simulink model "VehCtrl20260630_18B"  (R2018b)
settings: Solver=FixedStepAuto  StartTime=0.0  StopTime=inf  FixedStep=0.005  RelTol=1e-3
InitFcn:
  | mbd_mpc_consistency_checks(bdroot(gcs));
undefined symbols (not defined in the file): ANG_DEAD, BMS_NormalPwr, BrakeDeadZone, BrkPrsByBrkPct_TB_X, BrkPrsByBrkPct_TB_Y, DELAY_DISCHARGE, DELAY_RCUOFF, DRV_BACKWARD, DRV_BRAKE, DRV_FORWARD, DRV_NEUTRAL, DRV_PARK, DRV_UNPARK, DRV_ZEROTURN, EPB_LOCK, EPB_UNLOCK, ExtraLoadPwr, FanOff, fifo_0_vect, fifo_1_vect, HiFanReq, HV_finished, HV_No_Active, HV_POWER_OFF, HV_POWER_ON, HVDown, HVON, KaTLS_v_DrgUp_X_VehSpd, KeFTM_s_Way1OffDlyTime, KeFTM_TK_Way1CoolLv2OffBatTemp, KeFTM_TK_Way1CoolLv2OffMtrTemp, KeFTM_TK_Way1CoolLv2OnBatTemp, KeFTM_TK_Way1CoolLv2OnMtrTemp, KeFTM_TK_Way1CoolLv3OffBatTemp, KeFTM_TK_Way1CoolLv3OffMtrTemp, KeFTM_TK_Way1CoolLv3OnBatTemp, KeFTM_TK_Way1CoolLv3OnMtrTemp, KeFTM_TK_Way1CoolLv4OffBatTemp, KeFTM_TK_Way1CoolLv4OffMtrTemp, KeFTM_TK_Way1CoolLv4OnBatTemp, KeFTM_TK_Way1CoolLv4OnMtrTemp, Kp1, Kp2, LowFanReq, LQFP, MtrCmdGainFL, MtrCmdGainFR, MtrCmdGainRL, MtrCmdGainRR, MtrPwrFactor_RCU, MtrPwrHighToMidThd, MtrPwrLowToMidThd, MtrPwrMidToHighThd, MtrPwrMidToLowThd, MtrTrqMax, PCT_DEAD, Precharge, PTO_1000, PTO_540, pts1_fifo_0_vect ... (+32)
libraries: mbd_mpc574x_ec_toolbox x175, simulink x110, canmsglib x70
(part 11 of 15)

== system VehCtrl20260630_18B/SigIn/CAN1/MCU2VCU_17/UNPACK ==
  ID : Inport
  data : Inport  Port=2
  length : Inport  Port=3
  timestamp : Inport  Port=4
  Action Port : ActionPort  ActionType=case
  Add : Sum
  Bus Creator : BusCreator  Inputs=7  OutDataTypeStr=Bus: CAN_MESSAGE_BUS  NonVirtualBus=on
  Bus Creator1 : BusCreator  Inputs=14
  CAN Unpack6 : canmsglib/CAN Unpack  CANdbFile=D:\VCU\VCU_AgriculturalMachinery_ChangChun\VCU_AgriculturalMachinery_260519_ChangChun\CAN协议0519\MCU\MCU_dbc.dbc  MsgList=MCU_VCU_PTO_1  MsgName=MCU_VCU_PTO_1  MsgIDType=Extended (29-bit identifier)  MsgIdentifier=201893876  MsgLength=8  SignalInfo=MCU_Canlife$60$4$1$2$1$0$1$0$0$15$#MCU_ContactorStatus$56$2$1$2$1$0$1$0$0$3$#MCU_Gear$58$2$1$2$1$0$1$0$0$3$#MCU_SpdEst$16$16$1$2$1$0$1$-32000$-32000$33535$#MCU_TrqEst$0$16$1$2$1$0$1.000000e-01$-3200$-3200$3.353500e+03$#MCU_WorkStatus$48$8$1$2$1$0$1$0$0$255$#MCU_nCurrent$32$16$1$2$1$0$1.000000e-01$-3200$-3200$3.353500e+03$#  NSignals=7  IDPort=off  TimestampPort=off  ErrorPort=off  RemotePort=off  LengthPort=off  StatusPort=off  StartBits=str2num('[int32(60);int32(56);int32(58);int32(16);int32(0);int32(48);int32(32)]')  SignalSizes=str2num('[int32(4);int32(2);int32(2);int32(16);int32(16);int32(8);int32(16)]')  ByteOrders=str2num('[int32(1);int32(1);int32(1);int32(1);int32(1);int32(1);int32(1)]')  DataTypes=str2num('[int32(2);int32(2);int32(2);int32(2);int32(2);int32(2);int32(2)]')  MultiplexTypes=str2num('[int32(1);int32(1);int32(1);int32(1);int32(1);int32(1);int32(1)]')  MultiplexValues=str2num('[double(0);double(0);double(0);double(0);double(0);double(0);double(0)]')  Factors=str2num('[double(1);double(1);double(1);double(1);double(1.000000e-01);double(1);double(1.000000e-01)]')  Offsets=str2num('[double(0);double(0);double(0);double(-32000);double(-3200);double(0);double(-3200)]')  Minimums=str2num('[double(0);double(0);double(0);double(-32000);double(-3200);double(0);double(-3200)]')  Maximums=str2num('[double(15);double(3);double(3);double(33535);double(3.353500e+03);double(255);double(3.353500e+03)]')  ApplyMinMax=off
      settings: SourceProductName=Simulink Real-Time  SourceProductBaseCode=XP  DataFormat=CANdb specified signals
  Constant : Constant  OutDataTypeStr=uint8
  Constant1 : Constant  OutDataTypeStr=uint8
  Constant4 : Constant  Value=0  OutDataTypeStr=uint8
  Constant5 : Constant  Value=0  OutDataTypeStr=uint8
  Data Store Read : DataStoreRead  DataStoreName=Cnt_MCU5_1
  Data Store Write : DataStoreWrite  DataStoreName=Cnt_MCU5_1
  Data Type Conversion{,1..4,14..15,17} (8 alike) : DataTypeConversion  OutDataTypeStr=uint8
  Data Type Conversion18 : DataTypeConversion  OutDataTypeStr=uint32
  Data Type Conversion19 : DataTypeConversion  OutDataTypeStr=double
  Data Type Conversion60 : DataTypeConversion  OutDataTypeStr=single
  Data Type Conversion61 : DataTypeConversion  OutDataTypeStr=single
  Data Type Conversion62 : DataTypeConversion  OutDataTypeStr=single
  Gain : Gain  Gain=-1
  Subsystem : Subsystem
  Message : Outport
  wires:
  Constant4/1 -> Data Type Conversion15/1
  length/1 -> Data Type Conversion14/1
  data/1 -> Bus Creator/7  "Data"
  Data Type Conversion18/1 -> Bus Creator/5  "ID"
  Constant1/1 -> Data Type Conversion/1
  Constant5/1 -> Data Type Conversion17/1
  ID/1 -> Data Type Conversion18/1
  Data Type Conversion19/1 -> Bus Creator/6  "Timestamp"
  timestamp/1 -> Data Type Conversion19/1
  Data Type Conversion17/1 -> Bus Creator/4  "Error"
  Bus Creator/1 -> CAN Unpack6/1  "CAN_Msg_In"
  Data Type Conversion/1 -> Bus Creator/1  "Extended"
  Data Type Conversion14/1 -> Bus Creator/2  "Length"
  Data Type Conversion15/1 -> Bus Creator/3  "Remote"
  Bus Creator1/1 -> Message/1
  Data Type Conversion60/1 -> Bus Creator1/5  "MCU_TrqEst"
  Data Type Conversion61/1 -> Gain/1
  Data Type Conversion62/1 -> Bus Creator1/6  "MCU_nCurrent"
  Data Type Conversion1/1 -> Bus Creator1/1  "MCU_Canlife"
  CAN Unpack6/6 -> Data Type Conversion2/1
  CAN Unpack6/1 -> Data Type Conversion1/1
  CAN Unpack6/5 -> Data Type Conversion60/1
  CAN Unpack6/4 -> Data Type Conversion61/1
  CAN Unpack6/7 -> Data Type Conversion62/1
  CAN Unpack6/2 -> Data Type Conversion3/1
  CAN Unpack6/3 -> Data Type Conversion4/1
  Data Type Conversion3/1 -> Bus Creator1/2  "MCU_ContactorStatus"
  Data Type Conversion4/1 -> Bus Creator1/3  "MCU_Gear"
  Gain/1 -> Bus Creator1/4  "MCU_SpdEst"
  Data Type Conversion2/1 -> Subsystem/1(WorkStatus)  "MCU_WorkStatus"
  Subsystem/1(StartORStop) -> Bus Creator1/7  "MCU_StartORStop"
  Subsystem/2(Discharge) -> Bus Creator1/8  "MCU_Discharge"
  Subsystem/3(Direction) -> Bus Creator1/9  "MCU_Direction"
  Subsystem/4(DrvORBrk) -> Bus Creator1/10  "MCU_DrvORBrk"
  Subsystem/5(Fault) -> Bus Creator1/11  "MCU_Fault"
  Subsystem/6(Ready) -> Bus Creator1/12  "MCU_Ready"
  Subsystem/7(Mode) -> Bus Creator1/13  "MCU_Mode"
  Subsystem/8(PWM) -> Bus Creator1/14  "MCU_PWM"
  Add/1 -> Data Store Write/1
  Data Store Read/1 -> Add/1
  Constant/1 -> Add/2

== system VehCtrl20260630_18B/SigIn/CAN1/MCU2VCU_18/UNPACK ==
  ID : Inport
  data : Inport  Port=2
  length : Inport  Port=3
  timestamp : Inport  Port=4
  Action Port : ActionPort  ActionType=case
  Add : Sum
  Bus Creator : BusCreator  Inputs=7  OutDataTypeStr=Bus: CAN_MESSAGE_BUS  NonVirtualBus=on
  Bus Creator1 : BusCreator  Inputs=5
  CAN Unpack6 : canmsglib/CAN Unpack  CANdbFile=D:\VCU\VCU_AgriculturalMachinery_ChangChun\CAN协议8.4\MCU\MCU_Sheet1.dbc  MsgList=MCU_VCU_PTO_2  MsgName=MCU_VCU_PTO_2  MsgIDType=Extended (29-bit identifier)  MsgIdentifier=201959412  MsgLength=8  SignalInfo=MCU_AC_Voltage$16$16$1$2$1$0$1.000000e-01$0$0$6.553500e+03$#MCU_DC_Voltage$0$16$1$2$1$0$1.000000e-01$0$0$6.553500e+03$#MCU_nAvailI$32$16$1$2$1$0$1.000000e-01$0$0$6.553500e+03$#MCU_nControllerTemp$48$8$1$2$1$0$1$-40$-40$215$#MCU_nMotorTemp$56$8$1$2$1$0$1$-40$-40$215$#  NSignals=5  IDPort=off  TimestampPort=off  ErrorPort=off  RemotePort=off  LengthPort=off  StatusPort=off  StartBits=str2num('[int32(16);int32(0);int32(32);int32(48);int32(56)]')  SignalSizes=str2num('[int32(16);int32(16);int32(16);int32(8);int32(8)]')  ByteOrders=str2num('[int32(1);int32(1);int32(1);int32(1);int32(1)]')  DataTypes=str2num('[int32(2);int32(2);int32(2);int32(2);int32(2)]')  MultiplexTypes=str2num('[int32(1);int32(1);int32(1);int32(1);int32(1)]')  MultiplexValues=str2num('[double(0);double(0);double(0);double(0);double(0)]')  Factors=str2num('[double(1.000000e-01);double(1.000000e-01);double(1.000000e-01);double(1);double(1)]')  Offsets=str2num('[double(0);double(0);double(0);double(-40);double(-40)]')  Minimums=str2num('[double(0);double(0);double(0);double(-40);double(-40)]')  Maximums=str2num('[double(6.553500e+03);double(6.553500e+03);double(6.553500e+03);double(215);double(215)]')  ApplyMinMax=off
      settings: SourceProductName=Simulink Real-Time  SourceProductBaseCode=XP  DataFormat=CANdb specified signals
  Constant : Constant  OutDataTypeStr=uint8
  Constant1 : Constant  OutDataTypeStr=uint8
  Constant4 : Constant  Value=0  OutDataTypeStr=uint8
  Constant5 : Constant  Value=0  OutDataTypeStr=uint8
  Data Store Read : DataStoreRead  DataStoreName=Cnt_MCU5_2
  Data Store Write : DataStoreWrite  DataStoreName=Cnt_MCU5_2
  Data Store Write1 : DataStoreWrite  DataStoreName=PtoMotorTemp
  Data Store Write2 : DataStoreWrite  DataStoreName=PtoControlerTemp
  Data Type Conversion{,14..15,17} (4 alike) : DataTypeConversion  OutDataTypeStr=uint8
  Data Type Conversion{1,60..63} (5 alike) : DataTypeConversion  OutDataTypeStr=single
  Data Type Conversion18 : DataTypeConversion  OutDataTypeStr=uint32
  Data Type Conversion19 : DataTypeConversion  OutDataTypeStr=double
  Message : Outport
  wires:
  Constant4/1 -> Data Type Conversion15/1
  length/1 -> Data Type Conversion14/1
  data/1 -> Bus Creator/7  "Data"
  Data Type Conversion18/1 -> Bus Creator/5  "ID"
  Constant1/1 -> Data Type Conversion/1
  Constant5/1 -> Data Type Conversion17/1
  ID/1 -> Data Type Conversion18/1
  Data Type Conversion19/1 -> Bus Creator/6  "Timestamp"
  timestamp/1 -> Data Type Conversion19/1
  Data Type Conversion17/1 -> Bus Creator/4  "Error"
  Bus Creator/1 -> CAN Unpack6/1  "CAN_Msg_In"
  Data Type Conversion/1 -> Bus Creator/1  "Extended"
  Data Type Conversion14/1 -> Bus Creator/2  "Length"
  Data Type Conversion15/1 -> Bus Creator/3  "Remote"
  Bus Creator1/1 -> Message/1
  Data Type Conversion60/1 -> Bus Creator1/1  "MCU_DC_Voltage"
  Data Type Conversion61/1 -> Bus Creator1/2  "MCU_AC_Voltage"
  Data Type Conversion62/1 -> Bus Creator1/3  "MCU_nAvailI"
  Data Type Conversion63/1 -> Data Store Write2/1, Bus Creator1/4  "MCU_nControllerTemp"
  Data Type Conversion1/1 -> Data Store Write1/1, Bus Creator1/5  "MCU_nMotorTemp"
  CAN Unpack6/1 -> Data Type Conversion61/1  "MCU_FaultLevel"
  CAN Unpack6/2 -> Data Type Conversion60/1  "MCU_FaultNumber"
  CAN Unpack6/3 -> Data Type Conversion62/1
  CAN Unpack6/4 -> Data Type Conversion63/1
  CAN Unpack6/5 -> Data Type Conversion1/1
  Constant/1 -> Add/2
  Add/1 -> Data Store Write/1
  Data Store Read/1 -> Add/1

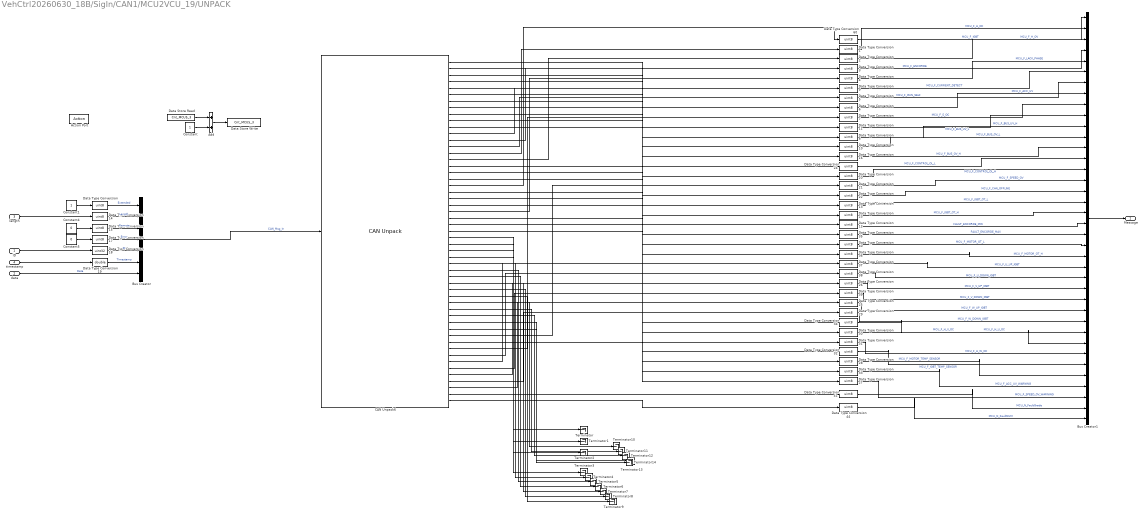
== system VehCtrl20260630_18B/SigIn/CAN1/MCU2VCU_19/UNPACK ==
  ID : Inport
  data : Inport  Port=2
  length : Inport  Port=3
  timestamp : Inport  Port=4
  Action Port : ActionPort  ActionType=case
  Add : Sum
  Bus Creator : BusCreator  Inputs=7  OutDataTypeStr=Bus: CAN_MESSAGE_BUS  NonVirtualBus=on
  Bus Creator1 : BusCreator  Inputs=38
  CAN Unpack6 : canmsglib/CAN Unpack  CANdbFile=D:\VCU\VCU_AgriculturalMachinery_ChangChun\CAN协议8.4\MCU\MCU_Sheet1.dbc  MsgList=MCU_VCU_PTO_3  MsgName=MCU_VCU_PTO_3  MsgIDType=Extended (29-bit identifier)  MsgIdentifier=202024948  MsgLength=8  SignalInfo=FAULT_ENCORDE_MAX$28$1$1$2$1$0$1$0$0$1$#FAULT_ENCORDE_MIN$27$1$1$2$1$0$1$0$0$1$#MCU_F_ACC_UV$11$1$1$2$1$0$1$0$0$1$#MCU_F_ACC_UV_WARNING$48$1$1$2$1$0$1$0$0$1$#MCU_F_BUS_OV_H$16$1$1$2$1$0$1$0$0$1$#MCU_F_BUS_OV_L$15$1$1$2$1$0$1$0$0$1$#MCU_F_BUS_UV_H$14$1$1$2$1$0$1$0$0$1$#MCU_F_BUS_UV_L$13$1$1$2$1$0$1$0$0$1$#MCU_F_CAN_OFFLINE$22$1$1$2$1$0$1$0$0$1$#MCU_F_CONTROL_OL_H$18$1$1$2$1$0$1$0$0$1$#MCU_F_CONTROL_OL_L$17$1$1$2$1$0$1$0$0$1$#MCU_F_CURRENT_DETECT$7$1$1$2$1$0$1$0$0$1$#MCU_F_ENCORDE$5$1$1$2$1$0$1$0$0$1$#MCU_F_GUN_SELF$10$1$1$2$1$0$1$0$0$1$#MCU_F_H_OC$1$1$1$2$1$0$1$0$0$1$#MCU_F_H_OV$3$1$1$2$1$0$1$0$0$1$#MCU_F_H_U_OC$42$1$1$2$1$0$1$0$0$1$#MCU_F_H_V_OC$43$1$1$2$1$0$1$0$0$1$#MCU_F_H_W_OC$44$1$1$2$1$0$1$0$0$1$#MCU_F_IGBT$0$1$1$2$1$0$1$0$0$1$#MCU_F_IGBT_OT_H$24$1$1$2$1$0$1$0$0$1$#MCU_F_IGBT_OT_L$23$1$1$2$1$0$1$0$0$1$#MCU_F_IGBT_TEMP_SENSOR$45$1$1$2$1$0$1$0$0$1$#MCU_F_LACK_PHASE$6$1$1$2$1$0$1$0$0$1$#MCU_F_MOTOR_OT_H$30$1$1$2$1$0$1$0$0$1$#MCU_F_MOTOR_OT_L$29$1$1$2$1$0$1$0$0$1$#MCU_F_MOTOR_TEMP_SENSOR$46$1$1$2$1$0$1$0$0$1$#MCU_F_RESERVE$2$1$1$2$1$0$1$0$0$1$#MCU_F_RESERVE$4$1$1$2$1$0$1$0$0$1$#MCU_F_RESERVE$8$1$1$2$1$0$1$0$0$1$#MCU_F_RESERVE$9$1$1$2$1$0$1$0$0$1$#MCU_F_RESERVE$19$1$1$2$1$0$1$0$0$1$#MCU_F_RESERVE$20$1$1$2$1$0$1$0$0$1$#MCU_F_RESERVE$25$1$1$2$1$0$1$0$0$1$#MCU_F_RESERVE$26$1$1$2$1$0$1$0$0$1$#MCU_F_RESERVE$31$1$1$2$1$0$1$0$0$1$#MCU_F_RESERVE$32$1$1$2$1$0$1$0$0$1$#MCU_F_RESERVE$33$1$1$2$1$0$1$0$0$1$#MCU_F_RESERVE$34$1$1$2$1$0$1$0$0$1$#MCU_F_RESERVE$41$1$1$2$1$0$1$0$0$1$#MCU_F_RESERVE$47$1$1$2$1$0$1$0$0$1$#MCU_F_RESERVE$50$1$1$2$1$0$1$0$0$1$#MCU_F_SPEED_OV$21$1$1$2$1$0$1$0$0$1$#MCU_F_SPEED_OV_WARNING$49$1$1$2$1$0$1$0$0$1$#MCU_F_S_OC$12$1$1$2$1$0$1$0$0$1$#MCU_F_U_DOWN_IGBT$36$1$1$2$1$0$1$0$0$1$#MCU_F_U_UP_IGBT$35$1$1$2$1$0$1$0$0$1$#MCU_F_V_DOWN_IGBT$38$1$1$2$1$0$1$0$0$1$#MCU_F_V_UP_IGBT$37$1$1$2$1$0$1$0$0$1$#MCU_F_W_DOWN_IGBT$40$1$1$2$1$0$1$0$0$1$#MCU_F_W_UP_IGBT$39$1$1$2$1$0$1$0$0$1$#MCU_N_FaultGrade$52$4$1$2$1$0$1$0$0$15$#MCU_N_FaultNUM$56$8$1$2$1$0$1$0$0$255$#  NSignals=53  IDPort=off  TimestampPort=off  ErrorPort=off  RemotePort=off  LengthPort=off  StatusPort=off  StartBits=str2num('[int32(28);int32(27);int32(11);int32(48);int32(16);int32(15);int32(14);int32(13);int32(22);int32(18);int32(17);int32(7);int32(5);int32(10);int32(1);int32(3);int32(42);int32(43);int32(44);int32(0);int32(24);int32(23);int32(45);int32(6);int32(30);int32(29);int32(46);int32(2);int32(4);int32(8);int32(9);int32(19);int32(20);int32(25);int32(26);int32(31);int32(32);int32(33);int32(34);int32(41);int32(47);int32(50);int32(21);int32(49);int32(12);int32(36);int32(35);int32(38);int32(37);int32(40);int32(39);int32(52);int32(56)]')  SignalSizes=str2num('[int32(1);int32(1);int32(1);int32(1);int32(1);int32(1);int32(1);int32(1);int32(1);int32(1);int32(1);int32(1);int32(1);int32(1);int32(1);int32(1);int32(1);int32(1);int32(1);int32(1);int32(1);int32(1);int32(1);int32(1);int32(1);int32(1);int32(1);int32(1);int32(1);int32(1);int32(1);int32(1);int32(1);int32(1);int32(1);int32(1);int32(1);int32(1);int32(1);int32(1);int32(1);int32(1);int32(1);int32(1);int32(1);int32(1);int32(1);int32(1);int32(1);int32(1);int32(1);int32(4);int32(8)]')  ByteOrders=str2num('[int32(1);int32(1);int32(1);int32(1);int32(1);int32(1);int32(1);int32(1);int32(1);int32(1);int32(1);int32(1);int32(1);int32(1);int32(1);int32(1);int32(1);int32(1);int32(1);int32(1);int32(1);int32(1);int32(1);int32(1);int32(1);int32(1);int32(1);int32(1);int32(1);int32(1);int32(1);int32(1);int32(1);int32(1);int32(1);int32(1);int32(1);int32(1);int32(1);int32(1);int32(1);int32(1);int32(1);int32(1);int32(1);int32(1);int32(1);int32(1);int32(1);int32(1);int32(1);int32(1);int32(1)]')  DataTypes=str2num('[int32(2);int32(2);int32(2);int32(2);int32(2);int32(2);int32(2);int32(2);int32(2);int32(2);int32(2);int32(2);int32(2);int32(2);int32(2);int32(2);int32(2);int32(2);int32(2);int32(2);int32(2);int32(2);int32(2);int32(2);int32(2);int32(2);int32(2);int32(2);int32(2);int32(2);int32(2);int32(2);int32(2);int32(2);int32(2);int32(2);int32(2);int32(2);int32(2);int32(2);int32(2);int32(2);int32(2);int32(2);int32(2);int32(2);int32(2);int32(2);int32(2);int32(2);int32(2);int32(2);int32(2)]')  MultiplexTypes=str2num('[int32(1);int32(1);int32(1);int32(1);int32(1);int32(1);int32(1);int32(1);int32(1);int32(1);int32(1);int32(1);int32(1);int32(1);int32(1);int32(1);int32(1);int32(1);int32(1);int32(1);int32(1);int32(1);int32(1);int32(1);int32(1);int32(1);int32(1);int32(1);int32(1);int32(1);int32(1);int32(1);int32(1);int32(1);int32(1);int32(1);int32(1);int32(1);int32(1);int32(1);int32(1);int32(1);int32(1);int32(1);int32(1);int32(1);int32(1);int32(1);int32(1);int32(1);int32(1);int32(1);int32(1)]')  MultiplexValues=str2num('[double(0);double(0);double(0);double(0);double(0);double(0);double(0);double(0);double(0);double(0);double(0);double(0);double(0);double(0);double(0);double(0);double(0);double(0);double(0);double(0);double(0);double(0);double(0);double(0);double(0);double(0);double(0);double(0);double(0);double(0);double(0);double(0);double(0);double(0);double(0);double(0);double(0);double(0);double(0);double(0);double(0);double(0);double(0);double(0);double(0);double(0);double(0);double(0);double(0);double(0);double(0);double(0);double(0)]')  Factors=str2num('[double(1);double(1);double(1);double(1);double(1);double(1);double(1);double(1);double(1);double(1);double(1);double(1);double(1);double(1);double(1);double(1);double(1);double(1);double(1);double(1);double(1);double(1);double(1);double(1);double(1);double(1);double(1);double(1);double(1);double(1);double(1);double(1);double(1);double(1);double(1);double(1);double(1);double(1);double(1);double(1);double(1);double(1);double(1);double(1);double(1);double(1);double(1);double(1);double(1);double(1);double(1);double(1);double(1)]')  Offsets=str2num('[double(0);double(0);double(0);double(0);double(0);double(0);double(0);double(0);double(0);double(0);double(0);double(0);double(0);double(0);double(0);double(0);double(0);double(0);double(0);double(0);double(0);double(0);double(0);double(0);double(0);double(0);double(0);double(0);double(0);double(0);double(0);double(0);double(0);double(0);double(0);double(0);double(0);double(0);double(0);double(0);double(0);double(0);double(0);double(0);double(0);double(0);double(0);double(0);double(0);double(0);double(0);double(0);double(0)]')  Minimums=str2num('[double(0);double(0);double(0);double(0);double(0);double(0);double(0);double(0);double(0);double(0);double(0);double(0);double(0);double(0);double(0);double(0);double(0);double(0);double(0);double(0);double(0);double(0);double(0);double(0);double(0);double(0);double(0);double(0);double(0);double(0);double(0);double(0);double(0);double(0);double(0);double(0);double(0);double(0);double(0);double(0);double(0);double(0);double(0);double(0);double(0);double(0);double(0);double(0);double(0);double(0);double(0);double(0);double(0)]')  Maximums=str2num('[double(1);double(1);double(1);double(1);double(1);double(1);double(1);double(1);double(1);double(1);double(1);double(1);double(1);double(1);double(1);double(1);double(1);double(1);double(1);double(1);double(1);double(1);double(1);double(1);double(1);double(1);double(1);double(1);double(1);double(1);double(1);double(1);double(1);double(1);double(1);double(1);double(1);double(1);double(1);double(1);double(1);double(1);double(1);double(1);double(1);double(1);double(1);double(1);double(1);double(1);double(1);double(15);double(255)]')  ApplyMinMax=off
      settings: SourceProductName=Simulink Real-Time  SourceProductBaseCode=XP  DataFormat=CANdb specified signals
  Constant : Constant  OutDataTypeStr=uint8
  Constant1 : Constant  OutDataTypeStr=uint8
  Constant4 : Constant  Value=0  OutDataTypeStr=uint8
  Constant5 : Constant  Value=0  OutDataTypeStr=uint8
  Data Store Read : DataStoreRead  DataStoreName=Cnt_MCU5_3
  Data Store Write : DataStoreWrite  DataStoreName=Cnt_MCU5_3
  Data Type Conversion{,1..17,20..41,44,60} (42 alike) : DataTypeConversion  OutDataTypeStr=uint8
  Data Type Conversion18 : DataTypeConversion  OutDataTypeStr=uint32
  Data Type Conversion19 : DataTypeConversion  OutDataTypeStr=double
  Terminator{,1..14} (15 alike) : Terminator
  Message : Outport
  wires:
  Data Type Conversion15/1 -> Bus Creator/3  "Remote"
  Data Type Conversion14/1 -> Bus Creator/2  "Length"
  Data Type Conversion/1 -> Bus Creator/1  "Extended"
  Data Type Conversion17/1 -> Bus Creator/4  "Error"
  timestamp/1 -> Data Type Conversion19/1
  Data Type Conversion19/1 -> Bus Creator/6  "Timestamp"
  ID/1 -> Data Type Conversion18/1
  Constant5/1 -> Data Type Conversion17/1
  Constant1/1 -> Data Type Conversion/1
  Data Type Conversion18/1 -> Bus Creator/5  "ID"
  data/1 -> Bus Creator/7  "Data"
  length/1 -> Data Type Conversion14/1
  Constant4/1 -> Data Type Conversion15/1
  Data Type Conversion13/1 -> Bus Creator1/18  "MCU_F_IGBT_OT_L"
  Data Type Conversion31/1 -> Bus Creator1/32  "MCU_F_H_W_OC"
  Data Type Conversion33/1 -> Bus Creator1/35  "MCU_F_ACC_UV_WARNING"
  Data Type Conversion27/1 -> Bus Creator1/36  "MCU_F_SPEED_OV_WARNING"
  Data Type Conversion38/1 -> Bus Creator1/25  "MCU_F_U_DOWN_IGBT"
  Bus Creator/1 -> CAN Unpack6/1  "CAN_Msg_In"
  Data Type Conversion23/1 -> Bus Creator1/19  "MCU_F_IGBT_OT_H"
  Data Type Conversion22/1 -> Bus Creator1/17  "MCU_F_CAN_OFFLINE"
  Data Type Conversion2/1 -> Bus Creator1/3  "MCU_F_H_OV"
  Data Type Conversion9/1 -> Bus Creator1/6  "MCU_F_CURRENT_DETECT"
  Data Type Conversion1/1 -> Bus Creator1/2  "MCU_F_H_OC"
  Data Type Conversion60/1 -> Bus Creator1/1  "MCU_F_IGBT"
  CAN Unpack6/29 -> Terminator1/1
  CAN Unpack6/46 -> Data Type Conversion38/1
  CAN Unpack6/52 -> Data Type Conversion41/1
  CAN Unpack6/41 -> Terminator13/1
  Data Type Conversion11/1 -> Bus Creator1/10  "MCU_F_BUS_UV_L"
  Data Type Conversion3/1 -> Bus Creator1/4  "MCU_F_ENCORDE"
  Data Type Conversion24/1 -> Bus Creator1/14  "MCU_F_CONTROL_OL_L"
  CAN Unpack6/7 -> Data Type Conversion8/1
  Data Type Conversion26/1 -> Bus Creator1/26  "MCU_F_V_UP_IGBT"
  CAN Unpack6/38 -> Terminator10/1
  CAN Unpack6/18 -> Data Type Conversion30/1
  CAN Unpack6/40 -> Terminator12/1
  CAN Unpack6/6 -> Data Type Conversion10/1
  CAN Unpack6/33 -> Terminator5/1
  Data Type Conversion28/1 -> Bus Creator1/34  "MCU_F_MOTOR_TEMP_SENSOR"
  Data Type Conversion4/1 -> Bus Creator1/5  "MCU_F_LACK_PHASE"
  CAN Unpack6/5 -> Data Type Conversion16/1
  Data Type Conversion36/1 -> Bus Creator1/23  "MCU_F_MOTOR_OT_H"
  CAN Unpack6/36 -> Terminator8/1
  CAN Unpack6/37 -> Terminator9/1
  CAN Unpack6/34 -> Terminator6/1
  CAN Unpack6/44 -> Data Type Conversion27/1
  CAN Unpack6/10 -> Data Type Conversion20/1
  Data Type Conversion34/1 -> Bus Creator1/30  "MCU_F_H_U_OC"
  Data Type Conversion12/1 -> Bus Creator1/20  "FAULT_ENCORDE_MIN"
  CAN Unpack6/31 -> Terminator3/1
  Data Type Conversion6/1 -> Bus Creator1/8  "MCU_F_ACC_UV"
  CAN Unpack6/50 -> Data Type Conversion29/1
  CAN Unpack6/51 -> Data Type Conversion25/1
  Data Type Conversion20/1 -> Bus Creator1/15  "MCU_F_CONTROL_OL_H"
  Data Type Conversion5/1 -> Bus Creator1/7  "MCU_F_GUN_SELF"
  Data Type Conversion25/1 -> Bus Creator1/28  "MCU_F_W_UP_IGBT"
  CAN Unpack6/21 -> Data Type Conversion23/1
  CAN Unpack6/25 -> Data Type Conversion36/1
  CAN Unpack6/26 -> Data Type Conversion40/1
  CAN Unpack6/42 -> Terminator14/1
  CAN Unpack6/28 -> Terminator/1
  Data Type Conversion40/1 -> Bus Creator1/22  "MCU_F_MOTOR_OT_L"
  CAN Unpack6/17 -> Data Type Conversion34/1
  CAN Unpack6/32 -> Terminator4/1
  CAN Unpack6/48 -> Data Type Conversion39/1
  CAN Unpack6/22 -> Data Type Conversion13/1
  Data Type Conversion7/1 -> Bus Creator1/9  "MCU_F_S_OC"
  Data Type Conversion32/1 -> Bus Creator1/33  "MCU_F_IGBT_TEMP_SENSOR"
  CAN Unpack6/43 -> Data Type Conversion21/1
  CAN Unpack6/14 -> Data Type Conversion5/1
  CAN Unpack6/47 -> Data Type Conversion37/1
  CAN Unpack6/3 -> Data Type Conversion6/1
  Data Type Conversion16/1 -> Bus Creator1/13  "MCU_F_BUS_OV_H"
  CAN Unpack6/20 -> Data Type Conversion60/1
  CAN Unpack6/19 -> Data Type Conversion31/1
  Data Type Conversion29/1 -> Bus Creator1/29  "MCU_F_W_DOWN_IGBT"
  Data Type Conversion41/1 -> Bus Creator1/37  "MCU_N_FaultGrade"
  CAN Unpack6/13 -> Data Type Conversion3/1
  CAN Unpack6/23 -> Data Type Conversion32/1
  CAN Unpack6/11 -> Data Type Conversion24/1
  Data Type Conversion39/1 -> Bus Creator1/27  "MCU_F_V_DOWN_IGBT"
  CAN Unpack6/27 -> Data Type Conversion28/1
  CAN Unpack6/45 -> Data Type Conversion7/1
  Data Type Conversion44/1 -> Bus Creator1/38  "MCU_N_FaultNUM"
  CAN Unpack6/9 -> Data Type Conversion22/1
  CAN Unpack6/30 -> Terminator2/1
  CAN Unpack6/8 -> Data Type Conversion11/1
  CAN Unpack6/1 -> Data Type Conversion35/1
  CAN Unpack6/16 -> Data Type Conversion2/1
  CAN Unpack6/35 -> Terminator7/1
  CAN Unpack6/24 -> Data Type Conversion4/1
  CAN Unpack6/4 -> Data Type Conversion33/1
  CAN Unpack6/49 -> Data Type Conversion26/1
  CAN Unpack6/2 -> Data Type Conversion12/1
  Data Type Conversion37/1 -> Bus Creator1/24  "MCU_F_U_UP_IGBT"
  CAN Unpack6/15 -> Data Type Conversion1/1
  Data Type Conversion35/1 -> Bus Creator1/21  "FAULT_ENCORDE_MAX"
  CAN Unpack6/53 -> Data Type Conversion44/1
  Data Type Conversion21/1 -> Bus Creator1/16  "MCU_F_SPEED_OV"
  Bus Creator1/1 -> Message/1
  CAN Unpack6/12 -> Data Type Conversion9/1
  CAN Unpack6/39 -> Terminator11/1
  Data Type Conversion8/1 -> Bus Creator1/11  "MCU_F_BUS_UV_H"
  Data Type Conversion10/1 -> Bus Creator1/12  "MCU_F_BUS_OV_L"
  Data Type Conversion30/1 -> Bus Creator1/31  "MCU_F_H_V_OC"
  Constant/1 -> Add/2
  Add/1 -> Data Store Write/1
  Data Store Read/1 -> Add/1

== system VehCtrl20260630_18B/SigIn/CAN1/MCU2VCU_2/UNPACK ==
  ID : Inport
  data : Inport  Port=2
  length : Inport  Port=3
  timestamp : Inport  Port=4
  Action Port : ActionPort  ActionType=case
  Add : Sum
  Bus Creator : BusCreator  Inputs=7  OutDataTypeStr=Bus: CAN_MESSAGE_BUS  NonVirtualBus=on
  Bus Creator1 : BusCreator  Inputs=5
  CAN Unpack6 : canmsglib/CAN Unpack  CANdbFile=D:\VCU\VCU_AgriculturalMachinery_ChangChun\CAN协议8.4\MCU\MCU_Sheet1.dbc  MsgList=MCU_VCU_FL_2  MsgName=MCU_VCU_FL_2  MsgIDType=Extended (29-bit identifier)  MsgIdentifier=201959411  MsgLength=8  SignalInfo=MCU_AC_Voltage$16$16$1$2$1$0$1.000000e-01$0$0$6.553500e+03$#MCU_DC_Voltage$0$16$1$2$1$0$1.000000e-01$0$0$6.553500e+03$#MCU_nAvailI$32$16$1$2$1$0$1.000000e-01$0$0$6.553500e+03$#MCU_nControllerTemp$48$8$1$2$1$0$1$-40$-40$215$#MCU_nMotorTemp$56$8$1$2$1$0$1$-40$-40$215$#  NSignals=5  IDPort=off  TimestampPort=off  ErrorPort=off  RemotePort=off  LengthPort=off  StatusPort=off  StartBits=str2num('[int32(16);int32(0);int32(32);int32(48);int32(56)]')  SignalSizes=str2num('[int32(16);int32(16);int32(16);int32(8);int32(8)]')  ByteOrders=str2num('[int32(1);int32(1);int32(1);int32(1);int32(1)]')  DataTypes=str2num('[int32(2);int32(2);int32(2);int32(2);int32(2)]')  MultiplexTypes=str2num('[int32(1);int32(1);int32(1);int32(1);int32(1)]')  MultiplexValues=str2num('[double(0);double(0);double(0);double(0);double(0)]')  Factors=str2num('[double(1.000000e-01);double(1.000000e-01);double(1.000000e-01);double(1);double(1)]')  Offsets=str2num('[double(0);double(0);double(0);double(-40);double(-40)]')  Minimums=str2num('[double(0);double(0);double(0);double(-40);double(-40)]')  Maximums=str2num('[double(6.553500e+03);double(6.553500e+03);double(6.553500e+03);double(215);double(215)]')  ApplyMinMax=off
      settings: SourceProductName=Simulink Real-Time  SourceProductBaseCode=XP  DataFormat=CANdb specified signals
  Constant : Constant  OutDataTypeStr=uint8
  Constant1 : Constant  OutDataTypeStr=uint8
  Constant4 : Constant  Value=0  OutDataTypeStr=uint8
  Constant5 : Constant  Value=0  OutDataTypeStr=uint8
  Data Store Read : DataStoreRead  DataStoreName=Cnt_MCU1_2
  Data Store Write : DataStoreWrite  DataStoreName=Cnt_MCU1_2
  Data Store Write2 : DataStoreWrite  DataStoreName=MtrMotorTempFL
  Data Store Write3 : DataStoreWrite  DataStoreName=MtrControlerTempFL
  Data Type Conversion{,14..15,17} (4 alike) : DataTypeConversion  OutDataTypeStr=uint8
  Data Type Conversion{1,60..63} (5 alike) : DataTypeConversion  OutDataTypeStr=single
  Data Type Conversion18 : DataTypeConversion  OutDataTypeStr=uint32
  Data Type Conversion19 : DataTypeConversion  OutDataTypeStr=double
  Message : Outport
  wires:
  Data Type Conversion1/1 -> Data Store Write2/1, Bus Creator1/5  "MCU_nMotorTemp"
  Data Type Conversion63/1 -> Data Store Write3/1, Bus Creator1/4  "MCU_nControllerTemp"
  Data Type Conversion62/1 -> Bus Creator1/3  "MCU_nAvailI"
  Data Type Conversion61/1 -> Bus Creator1/1  "MCU_AC_Voltage"
  Data Type Conversion60/1 -> Bus Creator1/2  "MCU_DC_Voltage"
  Bus Creator1/1 -> Message/1
  Data Type Conversion15/1 -> Bus Creator/3  "Remote"
  Data Type Conversion14/1 -> Bus Creator/2  "Length"
  Data Type Conversion/1 -> Bus Creator/1  "Extended"
  Bus Creator/1 -> CAN Unpack6/1  "CAN_Msg_In"
  Data Type Conversion17/1 -> Bus Creator/4  "Error"
  timestamp/1 -> Data Type Conversion19/1
  Data Type Conversion19/1 -> Bus Creator/6  "Timestamp"
  ID/1 -> Data Type Conversion18/1
  Constant5/1 -> Data Type Conversion17/1
  Constant1/1 -> Data Type Conversion/1
  Data Type Conversion18/1 -> Bus Creator/5  "ID"
  data/1 -> Bus Creator/7  "Data"
  length/1 -> Data Type Conversion14/1
  Constant4/1 -> Data Type Conversion15/1
  CAN Unpack6/1 -> Data Type Conversion61/1
  CAN Unpack6/2 -> Data Type Conversion60/1
  CAN Unpack6/3 -> Data Type Conversion62/1
  CAN Unpack6/4 -> Data Type Conversion63/1
  CAN Unpack6/5 -> Data Type Conversion1/1
  Constant/1 -> Add/2
  Data Store Read/1 -> Add/1
  Add/1 -> Data Store Write/1

== system VehCtrl20260630_18B/SigIn/CAN1/MCU2VCU_20/UNPACK ==
  ID : Inport
  data : Inport  Port=2
  length : Inport  Port=3
  timestamp : Inport  Port=4
  Action Port : ActionPort  ActionType=case
  Add : Sum
  Bus Creator : BusCreator  Inputs=7  OutDataTypeStr=Bus: CAN_MESSAGE_BUS  NonVirtualBus=on
  Bus Creator1 : BusCreator  Inputs=4
  CAN Unpack6 : canmsglib/CAN Unpack  CANdbFile=D:\VCU\VCU_AgriculturalMachinery_ChangChun\CAN协议8.4\MCU\MCU_Sheet1.dbc  MsgList=MCU_VCU_PTO_4  MsgName=MCU_VCU_PTO_4  MsgIDType=Extended (29-bit identifier)  MsgIdentifier=202090484  MsgLength=8  SignalInfo=MCU_MAX_BrakeTorque$16$16$1$2$1$0$1.000000e-01$0$0$6.553500e+03$#MCU_MAX_DriveTorque$0$16$1$2$1$0$1.000000e-01$0$0$6.553500e+03$#MCU_MAX_ForwardSpeed$32$16$1$2$1$0$1$0$0$65535$#MCU_MAX_ReverseSpeed$48$16$1$2$1$0$1$0$0$65535$#  NSignals=4  IDPort=off  TimestampPort=off  ErrorPort=off  RemotePort=off  LengthPort=off  StatusPort=off  StartBits=str2num('[int32(16);int32(0);int32(32);int32(48)]')  SignalSizes=str2num('[int32(16);int32(16);int32(16);int32(16)]')  ByteOrders=str2num('[int32(1);int32(1);int32(1);int32(1)]')  DataTypes=str2num('[int32(2);int32(2);int32(2);int32(2)]')  MultiplexTypes=str2num('[int32(1);int32(1);int32(1);int32(1)]')  MultiplexValues=str2num('[double(0);double(0);double(0);double(0)]')  Factors=str2num('[double(1.000000e-01);double(1.000000e-01);double(1);double(1)]')  Offsets=str2num('[double(0);double(0);double(0);double(0)]')  Minimums=str2num('[double(0);double(0);double(0);double(0)]')  Maximums=str2num('[double(6.553500e+03);double(6.553500e+03);double(65535);double(65535)]')  ApplyMinMax=off
      settings: SourceProductName=Simulink Real-Time  SourceProductBaseCode=XP  DataFormat=CANdb specified signals
  Constant : Constant  OutDataTypeStr=uint8
  Constant1 : Constant  OutDataTypeStr=uint8
  Constant4 : Constant  Value=0  OutDataTypeStr=uint8
  Constant5 : Constant  Value=0  OutDataTypeStr=uint8
  Data Store Read : DataStoreRead  DataStoreName=Cnt_MCU5_4
  Data Store Write : DataStoreWrite  DataStoreName=Cnt_MCU5_4
  Data Type Conversion{,14..15,17} (4 alike) : DataTypeConversion  OutDataTypeStr=uint8
  Data Type Conversion18 : DataTypeConversion  OutDataTypeStr=uint32
  Data Type Conversion19 : DataTypeConversion  OutDataTypeStr=double
  Data Type Conversion{60..63} (4 alike) : DataTypeConversion  OutDataTypeStr=single
  Message : Outport
  wires:
  Constant4/1 -> Data Type Conversion15/1
  length/1 -> Data Type Conversion14/1
  data/1 -> Bus Creator/7  "Data"
  Data Type Conversion18/1 -> Bus Creator/5  "ID"
  Constant1/1 -> Data Type Conversion/1
  Constant5/1 -> Data Type Conversion17/1
  ID/1 -> Data Type Conversion18/1
  Data Type Conversion19/1 -> Bus Creator/6  "Timestamp"
  timestamp/1 -> Data Type Conversion19/1
  Data Type Conversion17/1 -> Bus Creator/4  "Error"
  Bus Creator/1 -> CAN Unpack6/1  "CAN_Msg_In"
  Data Type Conversion/1 -> Bus Creator/1  "Extended"
  Data Type Conversion14/1 -> Bus Creator/2  "Length"
  Data Type Conversion15/1 -> Bus Creator/3  "Remote"
  Bus Creator1/1 -> Message/1
  Data Type Conversion60/1 -> Bus Creator1/1  "MCU_MAX_DriveTorque"
  Data Type Conversion61/1 -> Bus Creator1/2  "MCU_MAX_BrakeTorque"
  Data Type Conversion62/1 -> Bus Creator1/3  "MCU_MAX_ForwardSpeed"
  Data Type Conversion63/1 -> Bus Creator1/4  "MCU_MAX_ReverseSpeed"
  CAN Unpack6/1 -> Data Type Conversion61/1  "MCU_FaultLevel"
  CAN Unpack6/2 -> Data Type Conversion60/1  "MCU_FaultNumber"
  CAN Unpack6/3 -> Data Type Conversion62/1
  CAN Unpack6/4 -> Data Type Conversion63/1
  Constant/1 -> Add/2
  Add/1 -> Data Store Write/1
  Data Store Read/1 -> Add/1

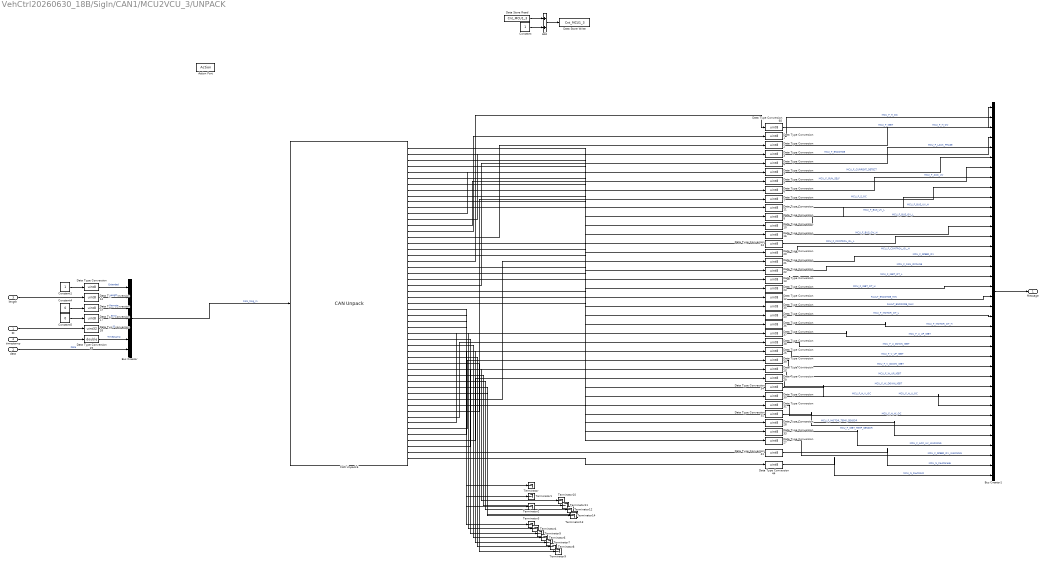
== system VehCtrl20260630_18B/SigIn/CAN1/MCU2VCU_3/UNPACK ==
  ID : Inport
  data : Inport  Port=2
  length : Inport  Port=3
  timestamp : Inport  Port=4
  Action Port : ActionPort  ActionType=case
  Add : Sum
  Bus Creator : BusCreator  Inputs=7  OutDataTypeStr=Bus: CAN_MESSAGE_BUS  NonVirtualBus=on
  Bus Creator1 : BusCreator  Inputs=38
  CAN Unpack6 : canmsglib/CAN Unpack  CANdbFile=D:\VCU\VCU_AgriculturalMachinery_ChangChun\CAN协议8.4\MCU\MCU_Sheet1.dbc  MsgList=MCU_VCU_FL_3  MsgName=MCU_VCU_FL_3  MsgIDType=Extended (29-bit identifier)  MsgIdentifier=202024947  MsgLength=8  SignalInfo=FAULT_ENCORDE_MAX$28$1$1$2$1$0$1$0$0$1$#FAULT_ENCORDE_MIN$27$1$1$2$1$0$1$0$0$1$#MCU_F_ACC_UV$11$1$1$2$1$0$1$0$0$1$#MCU_F_ACC_UV_WARNING$48$1$1$2$1$0$1$0$0$1$#MCU_F_BUS_OV_H$16$1$1$2$1$0$1$0$0$1$#MCU_F_BUS_OV_L$15$1$1$2$1$0$1$0$0$1$#MCU_F_BUS_UV_H$14$1$1$2$1$0$1$0$0$1$#MCU_F_BUS_UV_L$13$1$1$2$1$0$1$0$0$1$#MCU_F_CAN_OFFLINE$22$1$1$2$1$0$1$0$0$1$#MCU_F_CONTROL_OL_H$18$1$1$2$1$0$1$0$0$1$#MCU_F_CONTROL_OL_L$17$1$1$2$1$0$1$0$0$1$#MCU_F_CURRENT_DETECT$7$1$1$2$1$0$1$0$0$1$#MCU_F_ENCORDE$5$1$1$2$1$0$1$0$0$1$#MCU_F_GUN_SELF$10$1$1$2$1$0$1$0$0$1$#MCU_F_H_OC$1$1$1$2$1$0$1$0$0$1$#MCU_F_H_OV$3$1$1$2$1$0$1$0$0$1$#MCU_F_H_U_OC$42$1$1$2$1$0$1$0$0$1$#MCU_F_H_V_OC$43$1$1$2$1$0$1$0$0$1$#MCU_F_H_W_OC$44$1$1$2$1$0$1$0$0$1$#MCU_F_IGBT$0$1$1$2$1$0$1$0$0$1$#MCU_F_IGBT_OT_H$24$1$1$2$1$0$1$0$0$1$#MCU_F_IGBT_OT_L$23$1$1$2$1$0$1$0$0$1$#MCU_F_IGBT_TEMP_SENSOR$45$1$1$2$1$0$1$0$0$1$#MCU_F_LACK_PHASE$6$1$1$2$1$0$1$0$0$1$#MCU_F_MOTOR_OT_H$30$1$1$2$1$0$1$0$0$1$#MCU_F_MOTOR_OT_L$29$1$1$2$1$0$1$0$0$1$#MCU_F_MOTOR_TEMP_SENSOR$46$1$1$2$1$0$1$0$0$1$#MCU_F_RESERVE$2$1$1$2$1$0$1$0$0$1$#MCU_F_RESERVE$4$1$1$2$1$0$1$0$0$1$#MCU_F_RESERVE$8$1$1$2$1$0$1$0$0$1$#MCU_F_RESERVE$9$1$1$2$1$0$1$0$0$1$#MCU_F_RESERVE$19$1$1$2$1$0$1$0$0$1$#MCU_F_RESERVE$20$1$1$2$1$0$1$0$0$1$#MCU_F_RESERVE$25$1$1$2$1$0$1$0$0$1$#MCU_F_RESERVE$26$1$1$2$1$0$1$0$0$1$#MCU_F_RESERVE$31$1$1$2$1$0$1$0$0$1$#MCU_F_RESERVE$32$1$1$2$1$0$1$0$0$1$#MCU_F_RESERVE$33$1$1$2$1$0$1$0$0$1$#MCU_F_RESERVE$34$1$1$2$1$0$1$0$0$1$#MCU_F_RESERVE$41$1$1$2$1$0$1$0$0$1$#MCU_F_RESERVE$47$1$1$2$1$0$1$0$0$1$#MCU_F_RESERVE$50$1$1$2$1$0$1$0$0$1$#MCU_F_SPEED_OV$21$1$1$2$1$0$1$0$0$1$#MCU_F_SPEED_OV_WARNING$49$1$1$2$1$0$1$0$0$1$#MCU_F_S_OC$12$1$1$2$1$0$1$0$0$1$#MCU_F_U_DOWN_IGBT$36$1$1$2$1$0$1$0$0$1$#MCU_F_U_UP_IGBT$35$1$1$2$1$0$1$0$0$1$#MCU_F_V_DOWN_IGBT$38$1$1$2$1$0$1$0$0$1$#MCU_F_V_UP_IGBT$37$1$1$2$1$0$1$0$0$1$#MCU_F_W_DOWN_IGBT$40$1$1$2$1$0$1$0$0$1$#MCU_F_W_UP_IGBT$39$1$1$2$1$0$1$0$0$1$#MCU_N_FaultGrade$52$4$1$2$1$0$1$0$0$15$#MCU_N_FaultNUM$56$8$1$2$1$0$1$0$0$255$#  NSignals=53  IDPort=off  TimestampPort=off  ErrorPort=off  RemotePort=off  LengthPort=off  StatusPort=off  StartBits=str2num('[int32(28);int32(27);int32(11);int32(48);int32(16);int32(15);int32(14);int32(13);int32(22);int32(18);int32(17);int32(7);int32(5);int32(10);int32(1);int32(3);int32(42);int32(43);int32(44);int32(0);int32(24);int32(23);int32(45);int32(6);int32(30);int32(29);int32(46);int32(2);int32(4);int32(8);int32(9);int32(19);int32(20);int32(25);int32(26);int32(31);int32(32);int32(33);int32(34);int32(41);int32(47);int32(50);int32(21);int32(49);int32(12);int32(36);int32(35);int32(38);int32(37);int32(40);int32(39);int32(52);int32(56)]')  SignalSizes=str2num('[int32(1);int32(1);int32(1);int32(1);int32(1);int32(1);int32(1);int32(1);int32(1);int32(1);int32(1);int32(1);int32(1);int32(1);int32(1);int32(1);int32(1);int32(1);int32(1);int32(1);int32(1);int32(1);int32(1);int32(1);int32(1);int32(1);int32(1);int32(1);int32(1);int32(1);int32(1);int32(1);int32(1);int32(1);int32(1);int32(1);int32(1);int32(1);int32(1);int32(1);int32(1);int32(1);int32(1);int32(1);int32(1);int32(1);int32(1);int32(1);int32(1);int32(1);int32(1);int32(4);int32(8)]')  ByteOrders=str2num('[int32(1);int32(1);int32(1);int32(1);int32(1);int32(1);int32(1);int32(1);int32(1);int32(1);int32(1);int32(1);int32(1);int32(1);int32(1);int32(1);int32(1);int32(1);int32(1);int32(1);int32(1);int32(1);int32(1);int32(1);int32(1);int32(1);int32(1);int32(1);int32(1);int32(1);int32(1);int32(1);int32(1);int32(1);int32(1);int32(1);int32(1);int32(1);int32(1);int32(1);int32(1);int32(1);int32(1);int32(1);int32(1);int32(1);int32(1);int32(1);int32(1);int32(1);int32(1);int32(1);int32(1)]')  DataTypes=str2num('[int32(2);int32(2);int32(2);int32(2);int32(2);int32(2);int32(2);int32(2);int32(2);int32(2);int32(2);int32(2);int32(2);int32(2);int32(2);int32(2);int32(2);int32(2);int32(2);int32(2);int32(2);int32(2);int32(2);int32(2);int32(2);int32(2);int32(2);int32(2);int32(2);int32(2);int32(2);int32(2);int32(2);int32(2);int32(2);int32(2);int32(2);int32(2);int32(2);int32(2);int32(2);int32(2);int32(2);int32(2);int32(2);int32(2);int32(2);int32(2);int32(2);int32(2);int32(2);int32(2);int32(2)]')  MultiplexTypes=str2num('[int32(1);int32(1);int32(1);int32(1);int32(1);int32(1);int32(1);int32(1);int32(1);int32(1);int32(1);int32(1);int32(1);int32(1);int32(1);int32(1);int32(1);int32(1);int32(1);int32(1);int32(1);int32(1);int32(1);int32(1);int32(1);int32(1);int32(1);int32(1);int32(1);int32(1);int32(1);int32(1);int32(1);int32(1);int32(1);int32(1);int32(1);int32(1);int32(1);int32(1);int32(1);int32(1);int32(1);int32(1);int32(1);int32(1);int32(1);int32(1);int32(1);int32(1);int32(1);int32(1);int32(1)]')  MultiplexValues=str2num('[double(0);double(0);double(0);double(0);double(0);double(0);double(0);double(0);double(0);double(0);double(0);double(0);double(0);double(0);double(0);double(0);double(0);double(0);double(0);double(0);double(0);double(0);double(0);double(0);double(0);double(0);double(0);double(0);double(0);double(0);double(0);double(0);double(0);double(0);double(0);double(0);double(0);double(0);double(0);double(0);double(0);double(0);double(0);double(0);double(0);double(0);double(0);double(0);double(0);double(0);double(0);double(0);double(0)]')  Factors=str2num('[double(1);double(1);double(1);double(1);double(1);double(1);double(1);double(1);double(1);double(1);double(1);double(1);double(1);double(1);double(1);double(1);double(1);double(1);double(1);double(1);double(1);double(1);double(1);double(1);double(1);double(1);double(1);double(1);double(1);double(1);double(1);double(1);double(1);double(1);double(1);double(1);double(1);double(1);double(1);double(1);double(1);double(1);double(1);double(1);double(1);double(1);double(1);double(1);double(1);double(1);double(1);double(1);double(1)]')  Offsets=str2num('[double(0);double(0);double(0);double(0);double(0);double(0);double(0);double(0);double(0);double(0);double(0);double(0);double(0);double(0);double(0);double(0);double(0);double(0);double(0);double(0);double(0);double(0);double(0);double(0);double(0);double(0);double(0);double(0);double(0);double(0);double(0);double(0);double(0);double(0);double(0);double(0);double(0);double(0);double(0);double(0);double(0);double(0);double(0);double(0);double(0);double(0);double(0);double(0);double(0);double(0);double(0);double(0);double(0)]')  Minimums=str2num('[double(0);double(0);double(0);double(0);double(0);double(0);double(0);double(0);double(0);double(0);double(0);double(0);double(0);double(0);double(0);double(0);double(0);double(0);double(0);double(0);double(0);double(0);double(0);double(0);double(0);double(0);double(0);double(0);double(0);double(0);double(0);double(0);double(0);double(0);double(0);double(0);double(0);double(0);double(0);double(0);double(0);double(0);double(0);double(0);double(0);double(0);double(0);double(0);double(0);double(0);double(0);double(0);double(0)]')  Maximums=str2num('[double(1);double(1);double(1);double(1);double(1);double(1);double(1);double(1);double(1);double(1);double(1);double(1);double(1);double(1);double(1);double(1);double(1);double(1);double(1);double(1);double(1);double(1);double(1);double(1);double(1);double(1);double(1);double(1);double(1);double(1);double(1);double(1);double(1);double(1);double(1);double(1);double(1);double(1);double(1);double(1);double(1);double(1);double(1);double(1);double(1);double(1);double(1);double(1);double(1);double(1);double(1);double(15);double(255)]')  ApplyMinMax=off
      settings: SourceProductName=Simulink Real-Time  SourceProductBaseCode=XP  DataFormat=CANdb specified signals
  Constant : Constant  OutDataTypeStr=uint8
  Constant1 : Constant  OutDataTypeStr=uint8
  Constant4 : Constant  Value=0  OutDataTypeStr=uint8
  Constant5 : Constant  Value=0  OutDataTypeStr=uint8
  Data Store Read : DataStoreRead  DataStoreName=Cnt_MCU1_3
  Data Store Write : DataStoreWrite  DataStoreName=Cnt_MCU1_3
  Data Type Conversion{,1..17,20..41,44,60} (42 alike) : DataTypeConversion  OutDataTypeStr=uint8
  Data Type Conversion18 : DataTypeConversion  OutDataTypeStr=uint32
  Data Type Conversion19 : DataTypeConversion  OutDataTypeStr=double
  Terminator{,1..14} (15 alike) : Terminator
  Message : Outport
  wires:
  Constant4/1 -> Data Type Conversion15/1
  length/1 -> Data Type Conversion14/1
  data/1 -> Bus Creator/7  "Data"
  Data Type Conversion18/1 -> Bus Creator/5  "ID"
  Constant1/1 -> Data Type Conversion/1
  Constant5/1 -> Data Type Conversion17/1
  ID/1 -> Data Type Conversion18/1
  Data Type Conversion19/1 -> Bus Creator/6  "Timestamp"
  timestamp/1 -> Data Type Conversion19/1
  Data Type Conversion17/1 -> Bus Creator/4  "Error"
  Bus Creator/1 -> CAN Unpack6/1  "CAN_Msg_In"
  Data Type Conversion/1 -> Bus Creator/1  "Extended"
  Data Type Conversion14/1 -> Bus Creator/2  "Length"
  Data Type Conversion15/1 -> Bus Creator/3  "Remote"
  Bus Creator1/1 -> Message/1
  Data Type Conversion60/1 -> Bus Creator1/1  "MCU_F_IGBT"
  Data Type Conversion1/1 -> Bus Creator1/2  "MCU_F_H_OC"
  Data Type Conversion2/1 -> Bus Creator1/3  "MCU_F_H_OV"
  Data Type Conversion3/1 -> Bus Creator1/4  "MCU_F_ENCORDE"
  Data Type Conversion4/1 -> Bus Creator1/5  "MCU_F_LACK_PHASE"
  Data Type Conversion6/1 -> Bus Creator1/8  "MCU_F_ACC_UV"
  Data Type Conversion5/1 -> Bus Creator1/7  "MCU_F_GUN_SELF"
  Data Type Conversion9/1 -> Bus Creator1/6  "MCU_F_CURRENT_DETECT"
  Data Type Conversion11/1 -> Bus Creator1/10  "MCU_F_BUS_UV_L"
  Data Type Conversion8/1 -> Bus Creator1/11  "MCU_F_BUS_UV_H"
  Data Type Conversion10/1 -> Bus Creator1/12  "MCU_F_BUS_OV_L"
  Data Type Conversion7/1 -> Bus Creator1/9  "MCU_F_S_OC"
  Data Type Conversion22/1 -> Bus Creator1/17  "MCU_F_CAN_OFFLINE"
  Data Type Conversion12/1 -> Bus Creator1/20  "FAULT_ENCORDE_MIN"
  Data Type Conversion23/1 -> Bus Creator1/19  "MCU_F_IGBT_OT_H"
  Data Type Conversion13/1 -> Bus Creator1/18  "MCU_F_IGBT_OT_L"
  Data Type Conversion24/1 -> Bus Creator1/14  "MCU_F_CONTROL_OL_L"
  Data Type Conversion20/1 -> Bus Creator1/15  "MCU_F_CONTROL_OL_H"
  Data Type Conversion21/1 -> Bus Creator1/16  "MCU_F_SPEED_OV"
  Data Type Conversion16/1 -> Bus Creator1/13  "MCU_F_BUS_OV_H"
  Data Type Conversion29/1 -> Bus Creator1/29  "MCU_F_W_DOWN_IGBT"
  Data Type Conversion31/1 -> Bus Creator1/32  "MCU_F_H_W_OC"
  Data Type Conversion30/1 -> Bus Creator1/31  "MCU_F_H_V_OC"
  Data Type Conversion34/1 -> Bus Creator1/30  "MCU_F_H_U_OC"
  Data Type Conversion28/1 -> Bus Creator1/34  "MCU_F_MOTOR_TEMP_SENSOR"
  Data Type Conversion33/1 -> Bus Creator1/35  "MCU_F_ACC_UV_WARNING"
  Data Type Conversion27/1 -> Bus Creator1/36  "MCU_F_SPEED_OV_WARNING"
  Data Type Conversion32/1 -> Bus Creator1/33  "MCU_F_IGBT_TEMP_SENSOR"
  Data Type Conversion38/1 -> Bus Creator1/25  "MCU_F_U_DOWN_IGBT"
  Data Type Conversion25/1 -> Bus Creator1/28  "MCU_F_W_UP_IGBT"
  Data Type Conversion39/1 -> Bus Creator1/27  "MCU_F_V_DOWN_IGBT"
  Data Type Conversion26/1 -> Bus Creator1/26  "MCU_F_V_UP_IGBT"
  Data Type Conversion40/1 -> Bus Creator1/22  "MCU_F_MOTOR_OT_L"
  Data Type Conversion36/1 -> Bus Creator1/23  "MCU_F_MOTOR_OT_H"
  Data Type Conversion37/1 -> Bus Creator1/24  "MCU_F_U_UP_IGBT"
  Data Type Conversion35/1 -> Bus Creator1/21  "FAULT_ENCORDE_MAX"
  CAN Unpack6/52 -> Data Type Conversion41/1
  CAN Unpack6/53 -> Data Type Conversion44/1
  Data Type Conversion41/1 -> Bus Creator1/37  "MCU_N_FaultGrade"
  Data Type Conversion44/1 -> Bus Creator1/38  "MCU_N_FaultNUM"
  CAN Unpack6/1 -> Data Type Conversion35/1
  CAN Unpack6/2 -> Data Type Conversion12/1
  CAN Unpack6/5 -> Data Type Conversion16/1
  CAN Unpack6/6 -> Data Type Conversion10/1
  CAN Unpack6/7 -> Data Type Conversion8/1
  CAN Unpack6/8 -> Data Type Conversion11/1
  CAN Unpack6/9 -> Data Type Conversion22/1
  CAN Unpack6/10 -> Data Type Conversion20/1
  CAN Unpack6/11 -> Data Type Conversion24/1
  CAN Unpack6/12 -> Data Type Conversion9/1
  CAN Unpack6/13 -> Data Type Conversion3/1
  CAN Unpack6/15 -> Data Type Conversion1/1
  CAN Unpack6/16 -> Data Type Conversion2/1
  CAN Unpack6/17 -> Data Type Conversion34/1
  CAN Unpack6/18 -> Data Type Conversion30/1
  CAN Unpack6/19 -> Data Type Conversion31/1
  CAN Unpack6/20 -> Data Type Conversion60/1
  CAN Unpack6/21 -> Data Type Conversion23/1
  CAN Unpack6/22 -> Data Type Conversion13/1
  CAN Unpack6/23 -> Data Type Conversion32/1
  CAN Unpack6/14 -> Data Type Conversion5/1
  CAN Unpack6/24 -> Data Type Conversion4/1
  CAN Unpack6/26 -> Data Type Conversion40/1
  CAN Unpack6/44 -> Data Type Conversion27/1
  CAN Unpack6/43 -> Data Type Conversion21/1
  CAN Unpack6/45 -> Data Type Conversion7/1
  CAN Unpack6/46 -> Data Type Conversion38/1
  CAN Unpack6/47 -> Data Type Conversion37/1
  CAN Unpack6/48 -> Data Type Conversion39/1
  CAN Unpack6/49 -> Data Type Conversion26/1
  CAN Unpack6/51 -> Data Type Conversion25/1
  CAN Unpack6/50 -> Data Type Conversion29/1
  CAN Unpack6/4 -> Data Type Conversion33/1
  CAN Unpack6/3 -> Data Type Conversion6/1
  CAN Unpack6/25 -> Data Type Conversion36/1
  CAN Unpack6/27 -> Data Type Conversion28/1
  CAN Unpack6/28 -> Terminator/1
  CAN Unpack6/29 -> Terminator1/1
  CAN Unpack6/30 -> Terminator2/1
  CAN Unpack6/31 -> Terminator3/1
  CAN Unpack6/32 -> Terminator4/1
  CAN Unpack6/33 -> Terminator5/1
  CAN Unpack6/34 -> Terminator6/1
  CAN Unpack6/35 -> Terminator7/1
  CAN Unpack6/36 -> Terminator8/1
  CAN Unpack6/37 -> Terminator9/1
  CAN Unpack6/38 -> Terminator10/1
  CAN Unpack6/39 -> Terminator11/1
  CAN Unpack6/40 -> Terminator12/1
  CAN Unpack6/41 -> Terminator13/1
  CAN Unpack6/42 -> Terminator14/1
  Constant/1 -> Add/2
  Data Store Read/1 -> Add/1
  Add/1 -> Data Store Write/1

== system VehCtrl20260630_18B/SigIn/CAN1/MCU2VCU_4/UNPACK ==
  ID : Inport
  data : Inport  Port=2
  length : Inport  Port=3
  timestamp : Inport  Port=4
  Action Port : ActionPort  ActionType=case
  Add : Sum
  Bus Creator : BusCreator  Inputs=7  OutDataTypeStr=Bus: CAN_MESSAGE_BUS  NonVirtualBus=on
  Bus Creator1 : BusCreator  Inputs=4
  CAN Unpack6 : canmsglib/CAN Unpack  CANdbFile=D:\VCU\VCU_AgriculturalMachinery_ChangChun\CAN协议8.4\MCU\MCU_Sheet1.dbc  MsgList=MCU_VCU_FL_4  MsgName=MCU_VCU_FL_4  MsgIDType=Extended (29-bit identifier)  MsgIdentifier=202090483  MsgLength=8  SignalInfo=MCU_MAX_BrakeTorque$16$16$1$2$1$0$1.000000e-01$0$0$6.553500e+03$#MCU_MAX_DriveTorque$0$16$1$2$1$0$1.000000e-01$0$0$6.553500e+03$#MCU_MAX_ForwardSpeed$32$16$1$2$1$0$1$0$0$65535$#MCU_MAX_ReverseSpeed$48$16$1$2$1$0$1$0$0$65535$#  NSignals=4  IDPort=off  TimestampPort=off  ErrorPort=off  RemotePort=off  LengthPort=off  StatusPort=off  StartBits=str2num('[int32(16);int32(0);int32(32);int32(48)]')  SignalSizes=str2num('[int32(16);int32(16);int32(16);int32(16)]')  ByteOrders=str2num('[int32(1);int32(1);int32(1);int32(1)]')  DataTypes=str2num('[int32(2);int32(2);int32(2);int32(2)]')  MultiplexTypes=str2num('[int32(1);int32(1);int32(1);int32(1)]')  MultiplexValues=str2num('[double(0);double(0);double(0);double(0)]')  Factors=str2num('[double(1.000000e-01);double(1.000000e-01);double(1);double(1)]')  Offsets=str2num('[double(0);double(0);double(0);double(0)]')  Minimums=str2num('[double(0);double(0);double(0);double(0)]')  Maximums=str2num('[double(6.553500e+03);double(6.553500e+03);double(65535);double(65535)]')  ApplyMinMax=off
      settings: SourceProductName=Simulink Real-Time  SourceProductBaseCode=XP  DataFormat=CANdb specified signals
  Constant : Constant  OutDataTypeStr=uint8
  Constant1 : Constant  OutDataTypeStr=uint8
  Constant4 : Constant  Value=0  OutDataTypeStr=uint8
  Constant5 : Constant  Value=0  OutDataTypeStr=uint8
  Data Store Read : DataStoreRead  DataStoreName=Cnt_MCU1_4
  Data Store Write : DataStoreWrite  DataStoreName=Cnt_MCU1_4
  Data Type Conversion{,14..15,17} (4 alike) : DataTypeConversion  OutDataTypeStr=uint8
  Data Type Conversion18 : DataTypeConversion  OutDataTypeStr=uint32
  Data Type Conversion19 : DataTypeConversion  OutDataTypeStr=double
  Data Type Conversion{60..63} (4 alike) : DataTypeConversion  OutDataTypeStr=single
  Message : Outport
  wires:
  Data Type Conversion63/1 -> Bus Creator1/4  "MCU_MAX_ReverseSpeed"
  Data Type Conversion62/1 -> Bus Creator1/3  "MCU_MAX_ForwardSpeed"
  Data Type Conversion61/1 -> Bus Creator1/1  "MCU_MAX_BrakeTorque"
  Data Type Conversion60/1 -> Bus Creator1/2  "MCU_MAX_DriveTorque"
  Bus Creator1/1 -> Message/1
  Data Type Conversion15/1 -> Bus Creator/3  "Remote"
  Data Type Conversion14/1 -> Bus Creator/2  "Length"
  Data Type Conversion/1 -> Bus Creator/1  "Extended"
  Bus Creator/1 -> CAN Unpack6/1  "CAN_Msg_In"
  Data Type Conversion17/1 -> Bus Creator/4  "Error"
  timestamp/1 -> Data Type Conversion19/1
  Data Type Conversion19/1 -> Bus Creator/6  "Timestamp"
  ID/1 -> Data Type Conversion18/1
  Constant5/1 -> Data Type Conversion17/1
  Constant1/1 -> Data Type Conversion/1
  Data Type Conversion18/1 -> Bus Creator/5  "ID"
  data/1 -> Bus Creator/7  "Data"
  length/1 -> Data Type Conversion14/1
  Constant4/1 -> Data Type Conversion15/1
  CAN Unpack6/1 -> Data Type Conversion61/1
  CAN Unpack6/2 -> Data Type Conversion60/1
  CAN Unpack6/3 -> Data Type Conversion62/1
  CAN Unpack6/4 -> Data Type Conversion63/1
  Constant/1 -> Add/2
  Data Store Read/1 -> Add/1
  Add/1 -> Data Store Write/1
